simulink model "Verifica_LQG_20022026"  (R2025b)
settings: Solver=ode4  StartTime=0.0  StopTime=1e3  FixedStep=0.01  RelTol=1e-3
values from neighbouring files (symbols this model uses):
  A = double(subs(A_sym, p_eq_instabile, val_instabili))    [SvolgimentoEsame.m]
  B = double(subs(B_sym, p_eq_instabile, val_instabili))    [SvolgimentoEsame.m]
  C = eye(4)    [SvolgimentoEsame.m]
  D = zeros(4, 1)    [SvolgimentoEsame.m]
undefined symbols (not defined in the file or in its folder): A_kalman, B_kalman, C_kalman, C_LQR, D_kalman, K_LQR_x, r
libraries: simulink x2
settings Model: Creator=salvo  LastModifiedBy=salvo

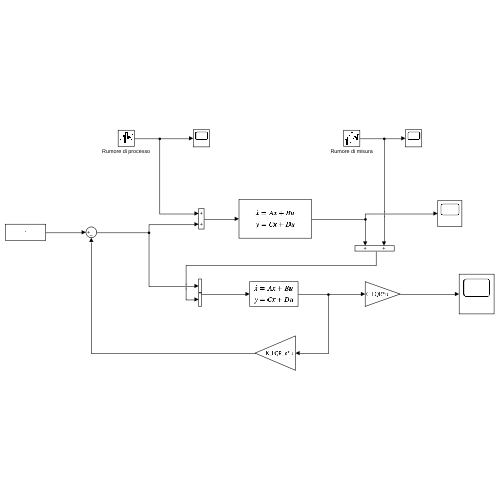
[thumbnail: Simulink's stored preview of the top-level diagram]
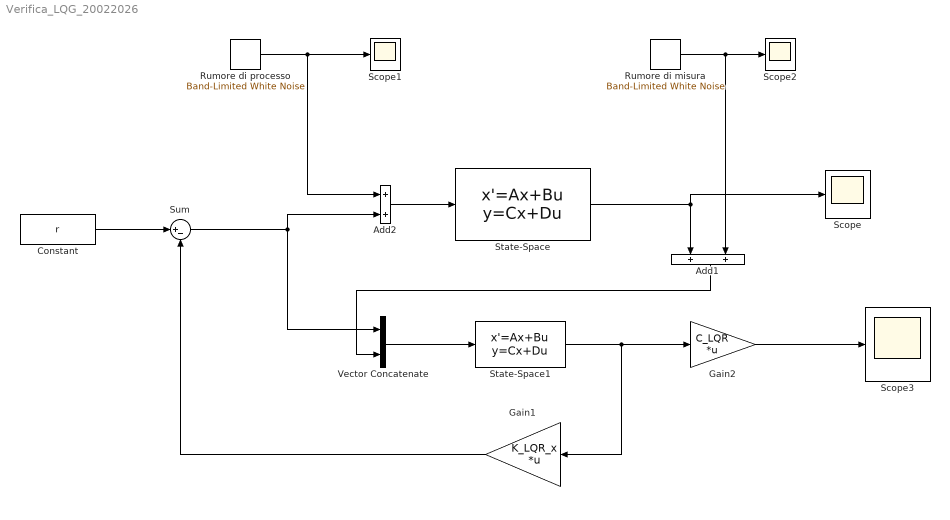
== system Verifica_LQG_20022026 ==
  Add1 : Sum
  Add2 : Sum
  Constant : Constant  Value=r
  Gain1 : Gain  Gain=K_LQR_x  Multiplication=Matrix(K*u)
  Gain2 : Gain  Gain=C_LQR  Multiplication=Matrix(K*u)
  Rumore di misura : simulink/Sources/Band-Limited White Noise  Cov=1  Ts=0.1  seed=[23341]
  Rumore di processo : simulink/Sources/Band-Limited White Noise  Cov=1  Ts=0.1  seed=[23341]
  Scope{,1..3} (4 alike) : Scope
      Scope settings: ActiveDisplayYMinimum=-2.0042813701226248  ActiveDisplayYMaximum=1.9552362050472611
      Scope1 settings: ActiveDisplayYMinimum=-1  ActiveDisplayYMaximum=1
      Scope2 settings: ActiveDisplayYMinimum=-1  ActiveDisplayYMaximum=1  DataLoggingVariableName=ScopeData2
      Scope3 settings: ActiveDisplayYMinimum=-5.8636128654195048  ActiveDisplayYMaximum=8.2253156794487623  DataLoggingVariableName=ScopeData3
  State-Space : StateSpace  A=A  B=B  C=C  D=D  InitialCondition=0
  State-Space1 : StateSpace  A=A_kalman  B=B_kalman  C=C_kalman  D=D_kalman  InitialCondition=0
  Sum : Sum  Inputs=|+-
  Vector Concatenate : Concatenate
  wires:
  Constant/1 -> Sum/1
  Sum/1 -> Add2/2, Vector Concatenate/1
  Rumore di processo/1 -> Add2/1, Scope1/1
  Rumore di misura/1 -> Scope2/1, Add1/2
  State-Space1/1 -> Gain1/1, Gain2/1
  State-Space/1 -> Scope/1, Add1/1
  Add2/1 -> State-Space/1
  Gain2/1 -> Scope3/1
  Vector Concatenate/1 -> State-Space1/1
  Add1/1 -> Vector Concatenate/2
  Gain1/1 -> Sum/2
